simulink model "example_PLL_IntegerN_model"  (R2024b)
settings: Solver=VariableStepAuto  StartTime=0.0  StopTime=10e-6  RelTol=1e-3
model workspace (MAT data in the model file):
  Frequency_14 = 50006354.387
  Frequency_20 = 0
  LockTime_29 = 0
  TargetFrequency_14 = 50000000
  TargetFrequency_20 = 2100000000
  TargetLockTime_29 = 3e-06
  TargetPhaseNoise_14 = [-85 -125 -150 -180]
  uniqueStringPll_14 = '38_0446'
  uniqueStringPll_20 = '60_1982'
  uniqueStringPll_29 = '23_478'
libraries: msbPllFoundation x5
settings Model: Creator=BrunoFraga  LastModifiedBy=BrunoFraga

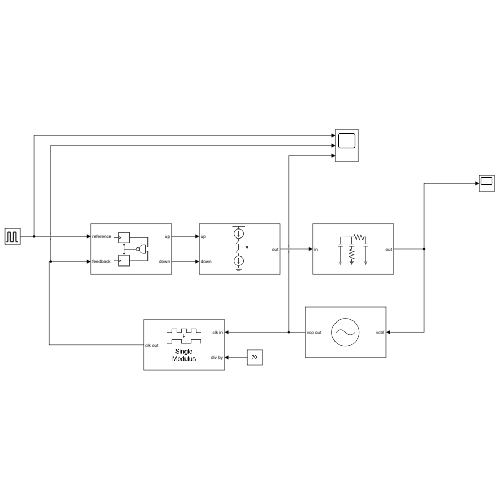
[thumbnail: Simulink's stored preview of the top-level diagram]
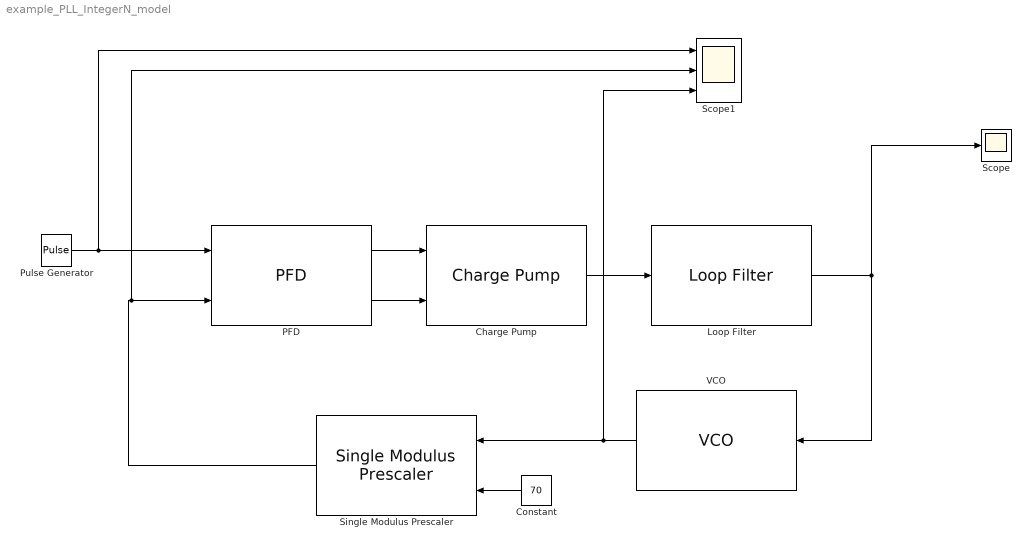
== system example_PLL_IntegerN_model ==
  Charge Pump : msbPllFoundation/Charge Pump  OutputCurrent=1e-3  InputThreshold=0.5  ExtraBuffer=off  NBuffer=1000  EnableCurrentImpairments=on  CurrentImbalance=1e-4  LeakageCurrent=1e-5  EnableTimingImpairments=on  DefaultOrAdvanced=Default  MaxFreqInterest=10e9  RiseFallUp=50e-12  PropDelayUp=60e-12  RiseFallDown=20e-12  PropDelayDown=40e-12
  Constant : Constant  Value=70
  Loop Filter : msbPllFoundation/Loop Filter  FilterType="3rd  order passive"  C1=13.1e-12  C2=144e-12  C3=0.941e-12  C4=1e-12  R2=1.33e3  R3=17e3  R4=12e3  ExtraBuffer=off  NBuffer=1000  EnableImpairments=off  Temperature=30
  PFD : msbPllFoundation/PFD  DeadbandCompensation=30e-12  ExtraBuffer=off  NBuffer=1000  EnableImpairments=on  DefaultOrAdvanced=Default  MaxFreqInterest=10e9  RiseFallTime=30e-12  PropDelay=50e-12
  Pulse Generator : DiscretePulseGenerator  PulseType=Time based  Period=1/30e6  PulseWidth=50
  Scope : Scope
  Scope1 : Scope  NumInputPorts=3
  Single Modulus Prescaler : msbPllFoundation/Single Modulus Prescaler  ExtraBuffer=off  NBuffer=1000
  VCO : msbPllFoundation/VCO  SpecifyUsing=Voltage sensitivity  Kvco=100e6  Fo=2.5e9  ControlVoltage=[-5 0 5]  OutputFrequency=[2e9 2.5e9 3e9]  Amplitude=1  ExtraBuffer=off  NBuffer=1000  AddPhaseNoise=off  Foffset=[30e3 100e3 1e6 3e6 10e6 100e6]  PhaseNoise=[-56 -106 -132 -143 -152 -172]  MaxKvco=100000000
  wires:
  Loop Filter/1 -> Scope/1, VCO/1
  Charge Pump/1 -> Loop Filter/1
  PFD/2 -> Charge Pump/2
  Single Modulus Prescaler/1 -> Scope1/2, PFD/2
  Constant/1 -> Single Modulus Prescaler/2
  PFD/1 -> Charge Pump/1
  Pulse Generator/1 -> Scope1/1, PFD/1
  VCO/1 -> Scope1/3, Single Modulus Prescaler/1
